simulink model "Bioreactor_FuzzyController_SimulinkBlock"  (R2016a)
settings: Solver=VariableStepAuto  SolverMode=SingleTasking  StartTime=0.0  StopTime=10.0  RelTol=1e-3
libraries: fuzblock x1
settings Model: Creator=saifu  LastModifiedBy=User
settings DataIOCC: ReturnWorkspaceOutputs=on
settings DebuggingCC: SFUnexpectedBacktrackingDiag=error  SFNoUnconditionalDefaultTransitionDiag=error
settings SFSimCC: SimUseLocalCustomCode=on
settings RTWCC: RTWUseLocalCustomCode=on
settings GRTTargetCC: TargetLangStandard=C99 (ISO)  GeneratePreprocessorConditionals=Use local settings
settings ConfigComp: CovMetricSettings=dwe  CovHtmlReporting=off  CovSaveCumulativeToWorkspaceVar=off  CovSaveSingleToWorkspaceVar=off  CovExternalEMLEnable=on

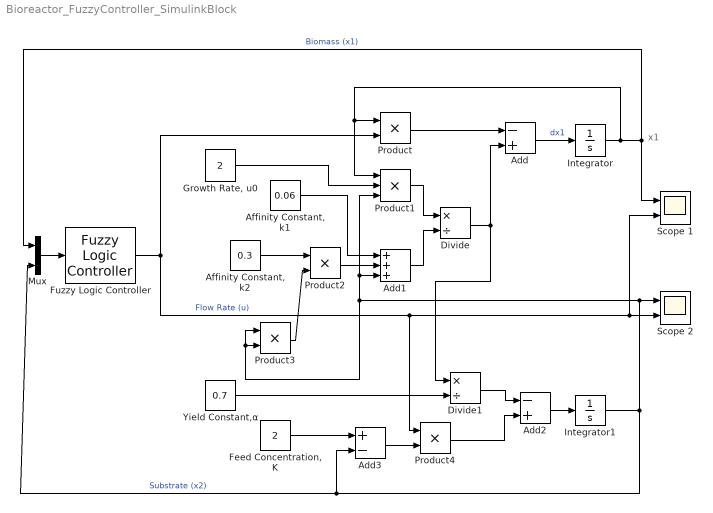
== system Bioreactor_FuzzyController_SimulinkBlock ==
  note: x1
  Add : Sum  Inputs=-+
  Add1 : Sum  Inputs=+++
  Add2 : Sum  Inputs=-+
  Add3 : Sum  Inputs=+-
  "Affinity Constant, k1" : Constant  Value=0.06
  "Affinity Constant, k2" : Constant  Value=0.3
  Divide : Product  Inputs=*/
  Divide1 : Product  Inputs=*/
  "Feed Concentration, K" : Constant  Value=2
  Fuzzy Logic Controller : fuzblock/Fuzzy Logic  Controller  fis=Bioreactor_fuzzy_controller
  "Growth Rate, u0" : Constant  Value=2  SampleTime=-1
  Integrator : Integrator
  Integrator1 : Integrator
  Mux : Mux  Inputs=2
  Product{,2..4} (4 alike) : Product
  Product1 : Product  Inputs=3
  Scope 1 : Scope  NumInputPorts=2
  Scope 2 : Scope  NumInputPorts=2
  "Yield Constant,α " : Constant  Value=0.7
  wires:
  Add/1 -> Integrator/1  "dx1"
  Divide/1 -> Add/2, Divide1/1
  Product/1 -> Add/1
  Product1/1 -> Divide/1
  Add1/1 -> Divide/2
  "Growth Rate, u0"/1 -> Product1/2
  Integrator1/1 -> Mux/2, Add3/2, Scope 2/1, Product3/2, Product3/1, Product1/3, Add1/3  "Substrate (x2)"
  Add2/1 -> Integrator1/1
  "Affinity Constant, k2"/1 -> Product2/1
  "Affinity Constant, k1"/1 -> Add1/1
  Product2/1 -> Add1/2
  "Feed Concentration, K"/1 -> Add3/1
  Add3/1 -> Product4/2
  "Yield Constant,α "/1 -> Divide1/2
  Divide1/1 -> Add2/1
  Product4/1 -> Add2/2
  Product3/1 -> Product2/2
  Integrator/1 -> Product/1, Product1/1, Mux/1, Scope 1/1  "Biomass (x1)"
  Mux/1 -> Fuzzy Logic Controller/1
  Fuzzy Logic Controller/1 -> Product/2, Scope 1/2, Scope 2/2, Product4/1  "Flow Rate (u)"
